simulink model "ksp_zad19_1"  (Simulink 2.20)
settings: Solver=ode45  StartTime=0.0  StopTime=500.0  RelTol=1e-3  AbsTol=1e-6
libraries: PID_continous_block x1
settings Model: ConsistencyChecking=off  RTWPlaceOutputsASAP=off

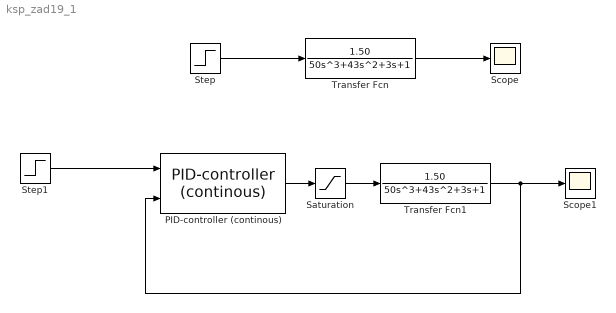
== system ksp_zad19_1 ==
  PID-controller (continous) : PID_continous_block/PID-controller (continous)  Description=PID_regulator  P=1.20  I=13  D=4
  Saturation : Saturate  UpperLimit=10  LowerLimit=0
  Scope : Scope
      settings: TickLabels=on  TimeRange=auto  YMin=-0.05  YMax=2.5  SaveToWorkspace=off  SaveName=ScopeData
  Scope1 : Scope
      settings: TickLabels=on  TimeRange=auto  YMin=-0.05  YMax=2.5  SaveToWorkspace=off  SaveName=ScopeData
  Step : Step  Time=0  Before=0  After=1
  Step1 : Step  Time=0  Before=0  After=1
  Transfer Fcn : TransferFcn  Numerator=[1.50]  Denominator=[50 43 3 1]
  Transfer Fcn1 : TransferFcn  Numerator=[1.50]  Denominator=[50 43 3 1]
  wires:
  Step/1 -> Transfer Fcn/1
  Transfer Fcn/1 -> Scope/1
  Step1/1 -> PID-controller (continous)/1
  Transfer Fcn1/1 -> Scope1/1, PID-controller (continous)/2
  PID-controller (continous)/1 -> Saturation/1
  Saturation/1 -> Transfer Fcn1/1
